simulink model "DeployableEMF"  (R2024a)
settings: Solver=FixedStepAuto  StartTime=0.0  StopTime=0  FixedStep=framePeriod_s  RelTol=1e-3
undefined symbols (not defined in the file): Aircraft, aircraftIC, AircraftModel, Avphi, DiscIntNeverNeededParam, EMF, EnableFF, EnableInputNoise, EnableRCHH, EnableSpeedHold, framePeriod_s, InitCond, Lv, Yv
libraries: simulink x14, simulink_extras x5
(part 1 of 2)
settings Model: Creator=zchen  LastModifiedBy=awalter
settings OptimizationCC: DefaultParameterBehavior=Inlined  GainParamInheritBuiltInType=on  UseFloatMulNetSlope=on  DefaultUnderspecifiedDataType=single  EnhancedBackFolding=on  PassReuseOutputArgsAs=Individual arguments  ZeroExternalMemoryAtStartup=off  ZeroInternalMemoryAtStartup=off  OptimizeBlockOrder=speed  DifferentSizesBufferReuse=on  OptimizationCustomize=off  EfficientTunableParamExpr=on
settings DebuggingCC: ParameterTunabilityLossMsg=error
settings HardwareCC: ProdLongLongMode=on
settings SFSimCC: MATLABDynamicMemAlloc=off
settings RTWCC: Description=Embedded Coder  SystemTargetFile=ert.tlc  GenCodeOnly=on  TemplateMakefile=ert_default_tmf  Toolchain=CMake  TargetLang=C++
settings CodeAppCC: ForceParamTrailComments=on  IgnoreCustomStorageClasses=off  OperatorAnnotations=on  SimulinkDataObjDesc=on  SFDataObjDesc=on  InsertBlockDesc=on
settings ERTTargetCC: TargetLangStandard=C++03 (ISO)  GenerateSampleERTMain=on  CodeInterfacePackaging=C++ class  InlinedParameterPlacement=NonHierarchical  RootIOFormat=Structure reference  ERTCustomFileTemplate=example_file_process.tlc

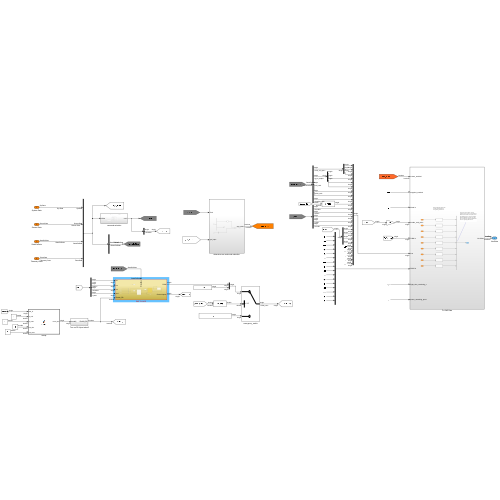
[thumbnail: Simulink's stored preview of the top-level diagram]
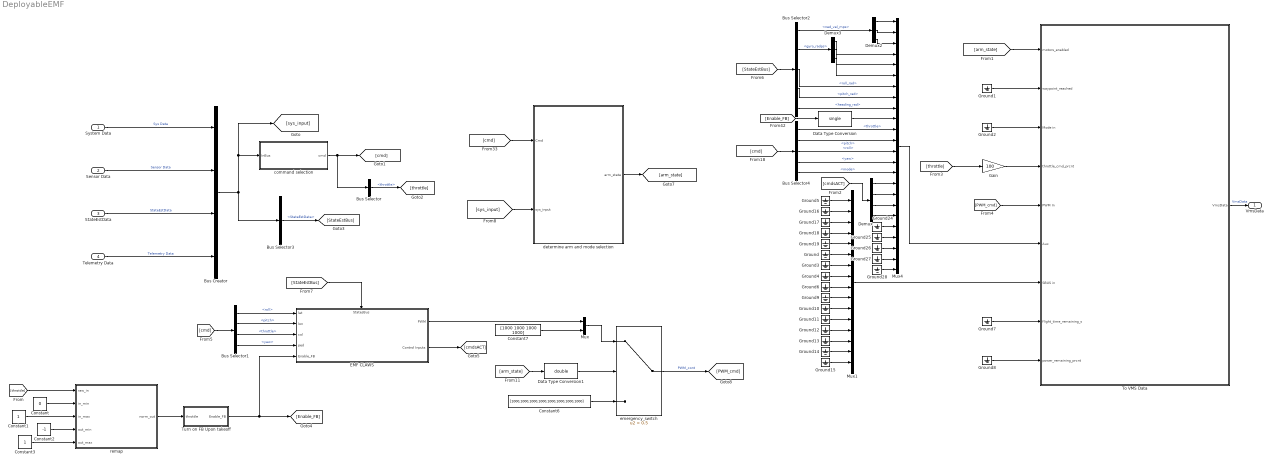
== system DeployableEMF ==
  System Data : Inport  OutDataTypeStr=Bus: SysData  SampleTime=framePeriod_s  BusOutputAsStruct=on
  Sensor Data : Inport  Port=2  OutDataTypeStr=Bus: SensorData  SampleTime=framePeriod_s  BusOutputAsStruct=on
  StateEstData : Inport  Port=3  OutDataTypeStr=Bus: StateEstData  SampleTime=framePeriod_s  BusOutputAsStruct=on
  Telemetry Data : Inport  Port=4  OutDataTypeStr=Bus: TelemData  SampleTime=framePeriod_s  BusOutputAsStruct=on
  Bus Creator : BusCreator  Inputs=4
  Bus Selector : BusSelector  OutputSignals=throttle
  Bus Selector1 : BusSelector  OutputSignals=roll,pitch,throttle,yaw
  Bus Selector2 : BusSelector  OutputSignals=bfs_ins.ned_vel_mps,bfs_ins.gyro_radps,bfs_ins.roll_rad,bfs_ins.pitch_rad,bfs_ins.heading_rad
  Bus Selector3 : BusSelector  OutputSignals=StateEstData
  Bus Selector4 : BusSelector  OutputSignals=throttle,pitch,roll,yaw,mode
  Constant : Constant  Value=0
  Constant1 : Constant
  Constant2 : Constant  Value=-1
  Constant3 : Constant
  Constant6 : Constant  Value=[1000,1000,1000,1000,1000,1000,1000,1000]  OutDataTypeStr=single
  Constant7 : Constant  Value=[1000 1000 1000 1000]  OutDataTypeStr=single
  Data Type Conversion : DataTypeConversion  OutDataTypeStr=single  SaturateOnIntegerOverflow=off  RndMeth=Floor
  Data Type Conversion1 : DataTypeConversion  OutDataTypeStr=double  SaturateOnIntegerOverflow=off  RndMeth=Floor
  Demux : Demux
  Demux2 : Demux  Outputs=3
  Demux3 : Demux  Outputs=3
  EMF CLAWS : Subsystem
      settings: PortSchema="{\"entries\":[{\"content\":{\"sides\":[{\"content\":{\"connectorIds\":[\"In1\",\"In2\",\"In3\",\"In4\",\"In5\"]},\"type\":\"ConnectorPlacement.EquallySpacedRectSide\",\"uuid\":\"fb2bd7fd-d988-4e33-8730-8c0f6eaa6827\"},{\"content\":{\"connectorIds\":[\"Out1\",\"Out2\"],\"side\":\"RIGHT\"},\"type\":\"ConnectorPlacement.EquallySpacedRectSide\",\"uuid\":\"7a7bb2dd-1c11-4f43-b871-d3aa786085a8\"},{\"content\":{\"connectorIds\":[\"In6\"],\"side\":\"TOP\"},\"type\":\"ConnectorPlacement.EquallySpacedRectSide\",\"uuid\":\"ea8fcfc4-ca21-4a8a-b475-95b355c5bc73\"},{\"content\":{\"side\":\"BOTTOM\"},\"type\":\"ConnectorPlacement.EquallySpacedRectSide\",\"uuid\":\"ba97ba4c-5167-4599-b94e-9748a5e0c732\"}]},\"type\":\"ConnectorPlacement.EquallySpacedConnector\",\"uuid\":\"d90d9832-6a61-4ee8-a098-cbdde4b4061b\"}],\"packageUris\":[\"http://schema.mathworks.com/mf0/Connector/R2020b\"],\"version\":\"1.0\"}"
  Gain : Gain  Gain=100
  Ground{,1..19,24..28} (25 alike) : Ground
  Mux : Mux  Inputs=2
  Mux1 : Mux  Inputs=16
  Mux4 : Mux  Inputs=24
  To VMS Data : Subsystem
  Turn on FB Upon takeoff : Subsystem
  command selection : Subsystem
  determine arm and mode selection : Subsystem
  emergency_switch : Switch  Criteria=u2 > Threshold  Threshold=0.5  SaturateOnIntegerOverflow=off  InputSameDT=off
  remap : MATLAB Function  TreatAsAtomicUnit=on
  VmsData : Outport  OutDataTypeStr=Bus: VmsData  SampleTime=framePeriod_s  BusOutputAsStruct=on
  wires:
  Turn on FB Upon takeoff/1(Enable_FB) -> [Enable_FB], EMF CLAWS/5(Enable_FB)
  Constant/1 -> remap/2(in_min)
  Ground7/1 -> To VMS Data/8(flight_time_remaining_s)
  [cmdsACT] -> Demux/1
  Ground/1 -> Mux1/6
  Bus Creator/1 -> Bus Selector3/1, [sys_input], command selection/1(InBus)
  Bus Selector1/3 -> EMF CLAWS/3(col)  "<throttle>"
  StateEstData/1 -> Bus Creator/3  "StateEstData"
  Mux4/1 -> To VMS Data/6(Aux)
  Bus Selector1/4 -> EMF CLAWS/4(ped)  "<yaw>"
  Ground14/1 -> Mux1/15
  Ground17/1 -> Mux1/3
  Bus Selector1/1 -> EMF CLAWS/1(lat)  "<roll>"
  Constant3/1 -> remap/5(out_max)
  Bus Selector1/2 -> EMF CLAWS/2(lon)  "<pitch>"
  [cmd] -> Bus Selector1/1
  determine arm and mode selection/1(arm_state) -> [arm_state]
  [arm_state] -> To VMS Data/1(motors_enabled)
  Ground1/1 -> To VMS Data/2(waypoint_reached)
  Bus Selector4/5 -> Mux4/15  "<mode>"
  [cmd] -> Bus Selector4/1
  Bus Selector4/4 -> Mux4/14  "<yaw>"
  [PWM_cmd] -> To VMS Data/5(PWM In)
  [Enable_FB] -> Data Type Conversion/1
  Ground9/1 -> Mux1/10
  Ground3/1 -> Mux1/7
  [throttle] -> Gain/1
  Ground16/1 -> Mux1/2
  Ground27/1 -> Mux4/23
  Ground28/1 -> Mux4/24
  Ground5/1 -> Mux1/1
  Demux/2 -> Mux4/17
  Ground4/1 -> Mux1/8
  command selection/1(cmd) -> Bus Selector/1, [cmd]
  Ground25/1 -> Mux4/21
  Constant1/1 -> remap/3(in_max)
  Data Type Conversion/1 -> Mux4/10
  Demux/4 -> Mux4/19
  Ground18/1 -> Mux1/4
  To VMS Data/1(VmsData) -> VmsData/1  "VmsData"
  EMF CLAWS/2(Control Inputs) -> [cmdsACT]
  Mux1/1 -> To VMS Data/7(SBUS in)
  Ground10/1 -> Mux1/11
  Ground19/1 -> Mux1/5
  Ground15/1 -> Mux1/16
  Demux/3 -> Mux4/18
  Bus Selector4/1 -> Mux4/11  "<throttle>"
  Ground2/1 -> To VMS Data/3(Mode in)
  Gain/1 -> To VMS Data/4(throttle_cmd_prcnt)
  Ground11/1 -> Mux1/12
  Bus Selector4/3 -> Mux4/13  "<roll>"
  System Data/1 -> Bus Creator/1  "Sys Data"
  [StateEstBus] -> EMF CLAWS/6(StatesBus)
  emergency_switch/1 -> [PWM_cmd]  "PWM_cont"
  Ground13/1 -> Mux1/14
  Telemetry Data/1 -> Bus Creator/4  "Telemetry Data"
  Constant2/1 -> remap/4(out_min)
  Data Type Conversion1/1 -> emergency_switch/2
  Constant7/1 -> Mux/2
  Demux/1 -> Mux4/16
  Ground8/1 -> To VMS Data/9(power_remaining_prcnt)
  Ground26/1 -> Mux4/22
  Bus Selector4/2 -> Mux4/12  "<pitch>"
  [cmd] -> determine arm and mode selection/1(Cmd)
  Ground6/1 -> Mux1/9
  [arm_state] -> Data Type Conversion1/1
  Sensor Data/1 -> Bus Creator/2  "Sensor Data"
  Ground24/1 -> Mux4/20
  Constant6/1 -> emergency_switch/3
  Bus Selector/1 -> [throttle]  "<throttle>"
  Mux/1 -> emergency_switch/1
  [throttle] -> remap/1(raw_in)
  Ground12/1 -> Mux1/13
  remap/1(norm_out) -> Turn on FB Upon takeoff/1(throttle)
  EMF CLAWS/1(PWM) -> Mux/1
  [sys_input] -> determine arm and mode selection/2(sys_input)
  Bus Selector3/1 -> [StateEstBus]  "<StateEstData>"
  Bus Selector2/5 -> Mux4/9  "<heading_rad>"
  Demux2/3 -> Mux4/3
  Bus Selector2/3 -> Mux4/7  "<roll_rad>"
  Demux2/2 -> Mux4/2
  Demux3/3 -> Mux4/6
  Demux2/1 -> Mux4/1
  Demux3/2 -> Mux4/5
  Demux3/1 -> Mux4/4
  Bus Selector2/1 -> Demux2/1  "<ned_vel_mps>"
  Bus Selector2/2 -> Demux3/1  "<gyro_radps>"
  [StateEstBus] -> Bus Selector2/1
  Bus Selector2/4 -> Mux4/8  "<pitch_rad>"

== system DeployableEMF/EMF CLAWS ==
  lat : Inport
  lon : Inport  Port=2
  col : Inport  Port=3
  ped : Inport  Port=4
  Enable_FB : Inport  Port=5
  StatesBus : Inport  Port=6
  ACAH Cmds & Spd Hold : Subsystem
      settings: PortSchema="{\"entries\":[{\"content\":{\"sides\":[{\"content\":{\"connectorIds\":[\"In1\",\"In2\"]},\"type\":\"ConnectorPlacement.EquallySpacedRectSide\",\"uuid\":\"c3aa03e9-ccb7-43c1-9798-8bf5432b2078\"},{\"content\":{\"connectorIds\":[\"Out1\",\"In3\"],\"side\":\"RIGHT\"},\"type\":\"ConnectorPlacement.EquallySpacedRectSide\",\"uuid\":\"89787a9d-9180-48b5-9998-cbe29e861495\"},{\"content\":{\"side\":\"TOP\"},\"type\":\"ConnectorPlacement.EquallySpacedRectSide\",\"uuid\":\"561bdc28-5c99-4c7e-b92e-eea3c95e9dce\"}]},\"type\":\"ConnectorPlacement.EquallySpacedConnector\",\"uuid\":\"f8321d21-0be0-47fc-a0ce-0477a72d6da9\"}],\"packageUris\":[\"http://schema.mathworks.com/mf0/Connector/R2020b\"],\"version\":\"1.0\"}"
  ACAH EMF1 : Subsystem
      settings: PortSchema="{\"entries\":[{\"content\":{\"sides\":[{\"content\":{\"connectorIds\":[\"In1\",\"In2\",\"In3\",\"In4\"]},\"type\":\"ConnectorPlacement.EquallySpacedRectSide\",\"uuid\":\"f0dc30a9-2643-4fce-a09e-da0b9dd6324b\"},{\"content\":{\"connectorIds\":[\"Out1\",\"Out2\",\"In5\"],\"side\":\"RIGHT\"},\"type\":\"ConnectorPlacement.EquallySpacedRectSide\",\"uuid\":\"f36ff2d8-c7c9-4ba3-92a3-b4ca37b19f9f\"},{\"content\":{\"side\":\"TOP\"},\"type\":\"ConnectorPlacement.EquallySpacedRectSide\",\"uuid\":\"7b352d47-5869-4cbf-a869-38e91cc0e44a\"},{\"content\":{\"side\":\"BOTTOM\"},\"type\":\"ConnectorPlacement.EquallySpacedRectSide\",\"uuid\":\"5fadfb50-1d15-4496-8b39-21c3867b197d\"}]},\"type\":\"ConnectorPlacement.EquallySpacedConnector\",\"uuid\":\"c5d3e032-086f-44da-ac5d-b4320e592dfa\"}],\"packageUris\":[\"http://schema.mathworks.com/mf0/Connector/R2020b\"],\"version\":\"1.0\"}"
  Mux : Mux
  PWM to Linear Model Inputs : Subsystem
  PWM : Outport
  Control Inputs : Outport  Port=2
  wires:
  StatesBus/1 -> ACAH Cmds & Spd Hold/3(StateEstBus), ACAH EMF1/4(StateEstBus)
  Mux/1 -> ACAH Cmds & Spd Hold/2(StickInputs), ACAH EMF1/1(cmdsStick)
  [Enable_FB] -> ACAH EMF1/2(Enable_FB)
  lat/1 -> Mux/1
  ACAH Cmds & Spd Hold/1(cmdsACAH) -> ACAH EMF1/3(cmdsACAH)
  [Enable_FB] -> ACAH Cmds & Spd Hold/1(Enable_FB)
  ped/1 -> Mux/4
  lon/1 -> Mux/2
  ACAH EMF1/1(PWM) -> PWM to Linear Model Inputs/1(PWM), PWM/1
  col/1 -> Mux/3
  Enable_FB/1 -> [Enable_FB]
  PWM to Linear Model Inputs/1(RotorSpeedsIn) -> ACAH EMF1/5(OmegasIn)
  ACAH EMF1/2(ControlInputs) -> Control Inputs/1

== system DeployableEMF/To VMS Data ==
  note: Cast to different data types to match with definition from global_definitions.h
  note: This is the bus creator. It acts similarly to the mux in Simulink but allows user match the inputs to the an arbitrary struct. This is useful to define interfaces. Check how this bus is matching with the VMS data struct in global_definitions.h
  motors_enabled : Inport
  waypoint_reached : Inport  Port=2
  Mode in : Inport  Port=3
  throttle_cmd_prcnt : Inport  Port=4
  PWM In : Inport  Port=5
  Aux : Inport  Port=6
  SBUS in : Inport  Port=7
  flight_time_remaining_s : Inport  Port=8
  power_remaining_prcnt : Inport  Port=9
  Bus Creator : BusCreator  Inputs=9  OutDataTypeStr=Bus: VmsData  NonVirtualBus=on
      settings: InheritFromInputs=off
  Cast : DataTypeConversion  OutDataTypeStr=int8  SaturateOnIntegerOverflow=off  RndMeth=Floor
  Cast To Boolean1 : DataTypeConversion  OutDataTypeStr=boolean  SaturateOnIntegerOverflow=off  RndMeth=Floor
  Cast To Boolean2 : DataTypeConversion  OutDataTypeStr=boolean  SaturateOnIntegerOverflow=off  RndMeth=Floor
  Cast To Single{,1..3} (4 alike) : DataTypeConversion  OutDataTypeStr=single  SaturateOnIntegerOverflow=off  RndMeth=Floor
  Cast1 : DataTypeConversion  OutDataTypeStr=int16  SaturateOnIntegerOverflow=off  RndMeth=Floor
  Cast2 : DataTypeConversion  OutDataTypeStr=int16  SaturateOnIntegerOverflow=off  RndMeth=Floor
  VmsData : Outport
  wires:
  Bus Creator/1 -> VmsData/1
  waypoint_reached/1 -> Cast To Boolean2/1  "advance_waypoint"
  motors_enabled/1 -> Cast To Boolean1/1  "motors_enabled"
  Mode in/1 -> Cast/1  "mode"
  SBUS in/1 -> Cast1/1  "sbus"
  PWM In/1 -> Cast2/1  "pwm"
  throttle_cmd_prcnt/1 -> Cast To Single1/1  "throttle_cmd_prcnt"
  Aux/1 -> Cast To Single3/1  "aux"
  Cast To Single2/1 -> Bus Creator/8  "power_remaining_prcnt"
  Cast To Single/1 -> Bus Creator/7  "flight_time_remaining_s"
  flight_time_remaining_s/1 -> Cast To Single/1  "flight_time_remaining_s"
  Cast To Boolean2/1 -> Bus Creator/1  "advance_waypoint"
  Cast To Boolean1/1 -> Bus Creator/2  "motors_enabled"
  Cast/1 -> Bus Creator/3  "mode"
  Cast1/1 -> Bus Creator/4  "sbus"
  Cast2/1 -> Bus Creator/5  "pwm"
  Cast To Single1/1 -> Bus Creator/6  "throttle_cmd_prcnt"
  power_remaining_prcnt/1 -> Cast To Single2/1  "power_remaining_prcnt"
  Cast To Single3/1 -> Bus Creator/9  "aux"

== system DeployableEMF/Turn on FB Upon takeoff ==
  throttle : Inport
  Constant3 : Constant
  Constant4 : Constant
  Constant5 : Constant  Value=0
  D Latch1 : simulink_extras/Flip Flops/D Latch
  Data Type Conversion2 : DataTypeConversion  SaturateOnIntegerOverflow=off  RndMeth=Floor
  Data Type Conversion3 : DataTypeConversion  SaturateOnIntegerOverflow=off  RndMeth=Floor
  Switch1 : Switch  Criteria=u2 > Threshold  Threshold=-0.2  SaturateOnIntegerOverflow=off  InputSameDT=off
  Terminator1 : Terminator
  Enable_FB : Outport
  wires:
  Constant4/1 -> Switch1/1
  Switch1/1 -> Data Type Conversion3/1
  D Latch1/1 -> Enable_FB/1
  throttle/1 -> Switch1/2
  Data Type Conversion3/1 -> D Latch1/2
  Constant3/1 -> Data Type Conversion2/1
  Data Type Conversion2/1 -> D Latch1/1
  D Latch1/2 -> Terminator1/1
  Constant5/1 -> Switch1/3

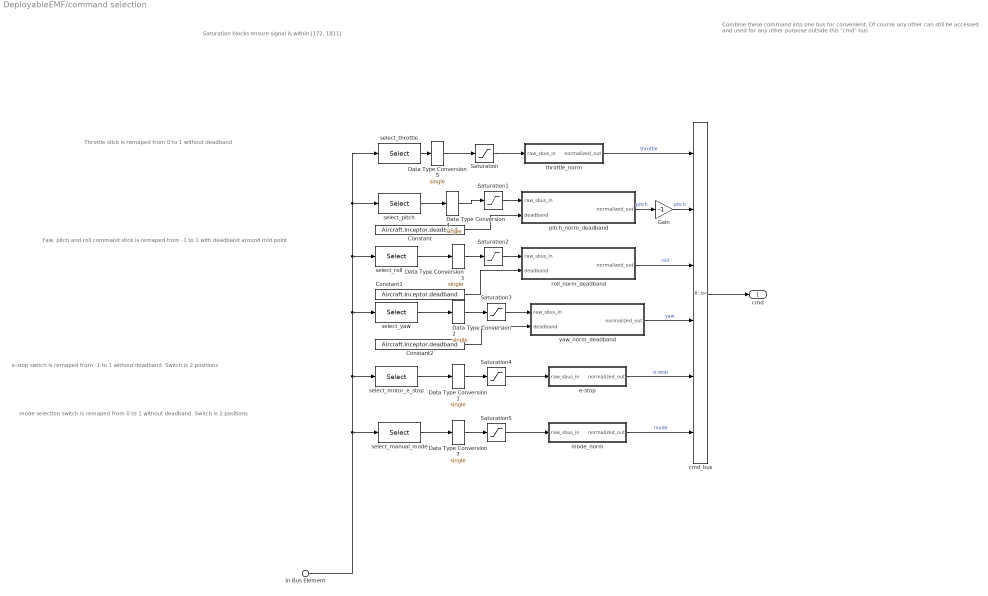
== system DeployableEMF/command selection ==
  note: Throttle stick is remaped from 0 to 1 without deadband
  note: Yaw, pitch and roll command stick is remaped from -1 to 1 with deadband around mid point
  note: e-stop switch is remaped from -1 to 1 without deadband. Switch is 2 positions
  note: mode selection switch is remaped from 0 to 1 without deadband. Switch is 2 positions
  note: Saturation blocks ensure signal is within [172, 1811]
  note: Combine these command into one bus for convenient. Of course any other can still be accessed and used for any other purpose outside this "cmd" bus
  In Bus Element : Inport  PortName=InBus  Element=Sensor Data.inceptor.ch
  Constant : Constant  Value=Aircraft.Inceptor.deadband  OutDataTypeStr=single
  Constant1 : Constant  Value=Aircraft.Inceptor.deadband  OutDataTypeStr=single
  Constant2 : Constant  Value=Aircraft.Inceptor.deadband  OutDataTypeStr=single
  Data Type Conversion{1..5,7} (6 alike) : DataTypeConversion  OutDataTypeStr=single  SaturateOnIntegerOverflow=off  RndMeth=Floor
  Gain : Gain  Gain=-1
  Saturation{,1..5} (6 alike) : Saturate  UpperLimit=1810  LowerLimit=174
  cmd_bus : BusCreator  Inputs=6
  e-stop : Subsystem
  mode_norm : Subsystem
  pitch_norm_deadband : Subsystem
  roll_norm_deadband : Subsystem
  select_manual_mode : Selector  IndexOptions=Index vector (dialog)  Indices=5  OutputSizes=1
  select_motor_e_stop : Selector  IndexOptions=Index vector (dialog)  Indices=8  OutputSizes=1
  select_pitch : Selector  IndexOptions=Index vector (dialog)  Indices=3  OutputSizes=1
  select_roll : Selector  IndexOptions=Index vector (dialog)  Indices=2  OutputSizes=1
  select_throttle : Selector  IndexOptions=Index vector (dialog)  Indices=1  OutputSizes=1
  select_yaw : Selector  IndexOptions=Index vector (dialog)  Indices=4  OutputSizes=1
  throttle_norm : Subsystem
  yaw_norm_deadband : Subsystem
  cmd : Outport
  wires:
  select_pitch/1 -> Data Type Conversion4/1
  select_yaw/1 -> Data Type Conversion2/1
  select_throttle/1 -> Data Type Conversion5/1
  cmd_bus/1 -> cmd/1
  Data Type Conversion5/1 -> Saturation/1
  select_roll/1 -> Data Type Conversion3/1
  Data Type Conversion1/1 -> Saturation4/1
  select_motor_e_stop/1 -> Data Type Conversion1/1
  Data Type Conversion7/1 -> Saturation5/1
  select_manual_mode/1 -> Data Type Conversion7/1
  Data Type Conversion2/1 -> Saturation3/1
  Constant2/1 -> yaw_norm_deadband/2(deadband)
  throttle_norm/1(normalized_out) -> cmd_bus/1  "throttle"
  roll_norm_deadband/1(normalized_out) -> cmd_bus/3  "roll"
  pitch_norm_deadband/1(normalized_out) -> Gain/1  "pitch"
  Data Type Conversion4/1 -> Saturation1/1
  Constant/1 -> pitch_norm_deadband/2(deadband)
  Constant1/1 -> roll_norm_deadband/2(deadband)
  Data Type Conversion3/1 -> Saturation2/1
  yaw_norm_deadband/1(normalized_out) -> cmd_bus/4  "yaw"
  e-stop/1(normalized_out) -> cmd_bus/5  "e-stop"
  mode_norm/1(normalized_out) -> cmd_bus/6  "mode"
  In Bus Element/1 -> select_roll/1, select_throttle/1, select_pitch/1, select_yaw/1, select_motor_e_stop/1, select_manual_mode/1
  Saturation/1 -> throttle_norm/1(raw_sbus_in)
  Saturation2/1 -> roll_norm_deadband/1(raw_sbus_in)
  Saturation3/1 -> yaw_norm_deadband/1(raw_sbus_in)
  Saturation4/1 -> e-stop/1(raw_sbus_in)
  Saturation5/1 -> mode_norm/1(raw_sbus_in)
  Saturation1/1 -> pitch_norm_deadband/1(raw_sbus_in)
  Gain/1 -> cmd_bus/2  "pitch"

== system DeployableEMF/determine arm and mode selection ==
  Cmd : Inport
  sys_input : Inport  Port=2
  AND : Logic  IconShape=distinctive  AllPortsSameDT=off  OutDataTypeStr=boolean
  Bus Selector : BusSelector  OutputSignals=StateEstData.bfs_ins.initialized
  Bus Selector1 : BusSelector  OutputSignals=mode,throttle
  Compare To Constant1 : simulink/Logic and Bit Operations/Compare To Constant  relop=>  const=0.5  OutDataTypeStr=boolean
  Terminator : Terminator
  arm_state : Outport
  wires:
  Cmd/1 -> Bus Selector1/1
  Bus Selector1/2 -> Terminator/1  "<throttle>"
  sys_input/1 -> Bus Selector/1
  Compare To Constant1/1 -> AND/1
  AND/1 -> arm_state/1
  Bus Selector1/1 -> Compare To Constant1/1  "<mode>"
  Bus Selector/1 -> AND/2  "<initialized>"

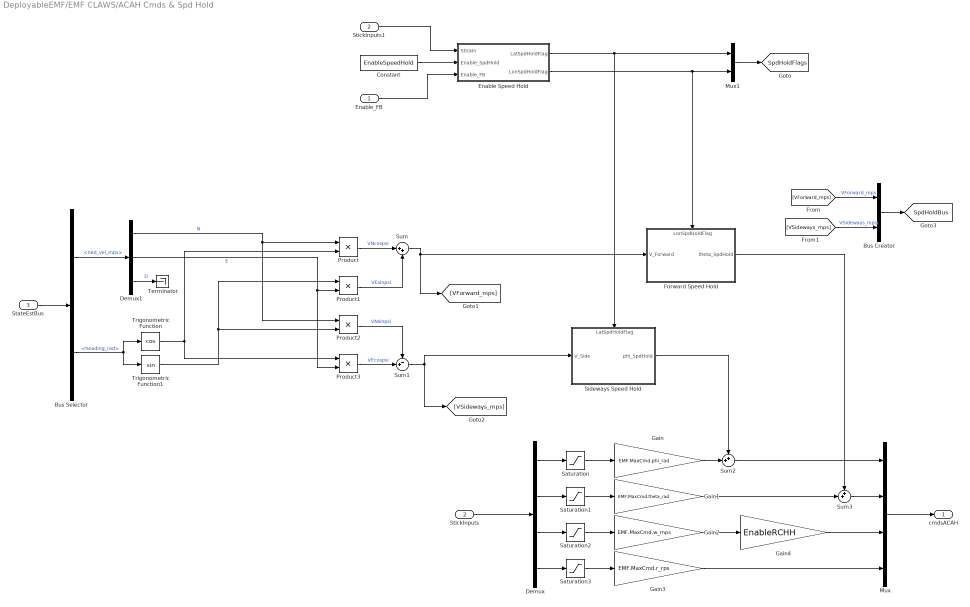
== system DeployableEMF/EMF CLAWS/ACAH Cmds & Spd Hold ==
  Enable_FB : Inport
  StickInputs : Inport  Port=2
  StateEstBus : Inport  Port=3
  Bus Creator : BusCreator  Inputs=2
  Bus Selector : BusSelector  OutputSignals=bfs_ins.ned_vel_mps,bfs_ins.heading_rad
  Constant : Constant  Value=EnableSpeedHold
  Demux : Demux
  Demux1 : Demux  Outputs=3
  Enable Speed Hold : Subsystem
  Forward Speed Hold : Subsystem
      settings: PortSchema="{\"entries\":[{\"content\":{\"sides\":[{\"content\":{\"connectorIds\":[\"In1\"]},\"type\":\"ConnectorPlacement.EquallySpacedRectSide\",\"uuid\":\"787a0d40-d54a-40fd-80f9-efd334690e34\"},{\"content\":{\"connectorIds\":[\"Out1\"],\"side\":\"RIGHT\"},\"type\":\"ConnectorPlacement.EquallySpacedRectSide\",\"uuid\":\"f6a8c8e2-752b-42ff-b4f2-32f20fdea40d\"},{\"content\":{\"connectorIds\":[\"In2\"],\"side\":\"TOP\"},\"type\":\"ConnectorPlacement.EquallySpacedRectSide\",\"uuid\":\"415bab51-e904-4948-b139-fad0363c569f\"},{\"content\":{\"side\":\"BOTTOM\"},\"type\":\"ConnectorPlacement.EquallySpacedRectSide\",\"uuid\":\"fe1710f6-98f7-4914-bba4-54f9a2ec34d8\"}]},\"type\":\"ConnectorPlacement.EquallySpacedConnector\",\"uuid\":\"a4ae154f-8926-4c51-a0ea-11671019ffb8\"}],\"packageUris\":[\"http://schema.mathworks.com/mf0/Connector/R2020b\"],\"version\":\"1.0\"}"
  Gain : Gain  Gain=EMF.MaxCmd.phi_rad
  Gain1 : Gain  Gain=EMF.MaxCmd.theta_rad
  Gain2 : Gain  Gain=EMF.MaxCmd.w_mps
  Gain3 : Gain  Gain=EMF.MaxCmd.r_rps
  Gain4 : Gain  Gain=EnableRCHH
  Mux : Mux
  Mux1 : Mux  Inputs=2
  Product{,1..3} (4 alike) : Product
  Saturation{,1..3} (4 alike) : Saturate  UpperLimit=1  LowerLimit=-1
  Sideways Speed Hold : Subsystem
      settings: PortSchema="{\"entries\":[{\"content\":{\"sides\":[{\"content\":{\"connectorIds\":[\"In1\"]},\"type\":\"ConnectorPlacement.EquallySpacedRectSide\",\"uuid\":\"787a0d40-d54a-40fd-80f9-efd334690e34\"},{\"content\":{\"connectorIds\":[\"Out1\"],\"side\":\"RIGHT\"},\"type\":\"ConnectorPlacement.EquallySpacedRectSide\",\"uuid\":\"f6a8c8e2-752b-42ff-b4f2-32f20fdea40d\"},{\"content\":{\"connectorIds\":[\"In2\"],\"side\":\"TOP\"},\"type\":\"ConnectorPlacement.EquallySpacedRectSide\",\"uuid\":\"415bab51-e904-4948-b139-fad0363c569f\"}]},\"type\":\"ConnectorPlacement.EquallySpacedConnector\",\"uuid\":\"a4ae154f-8926-4c51-a0ea-11671019ffb8\"}],\"packageUris\":[\"http://schema.mathworks.com/mf0/Connector/R2020b\"],\"version\":\"1.0\"}"
  StickInputs1 : InportShadow  Port=2
  Sum : Sum  Inputs=|++
  Sum1 : Sum  Inputs=-+|
  Sum2 : Sum  Inputs=++|
  Sum3 : Sum  Inputs=++|
  Terminator : Terminator
  Trigonometric Function : Trigonometry  Operator=cos
  Trigonometric Function1 : Trigonometry
  cmdsACAH : Outport
  tag scope: SpdHoldBus=global, SpdHoldFlags=global
  wires:
  Demux/1 -> Saturation/1
  Demux/2 -> Saturation1/1
  Demux/3 -> Saturation2/1
  Demux/4 -> Saturation3/1
  Saturation/1 -> Gain/1
  Saturation1/1 -> Gain1/1
  Saturation2/1 -> Gain2/1
  Saturation3/1 -> Gain3/1
  Gain2/1 -> Gain4/1
  Gain3/1 -> Mux/4
  Sum3/1 -> Mux/2
  Gain/1 -> Sum2/2
  StateEstBus/1 -> Bus Selector/1
  Mux/1 -> cmdsACAH/1
  StickInputs/1 -> Demux/1
  Demux1/1 -> Product/1, Product2/1  "N"
  Demux1/2 -> Product3/2, Product1/2  "E"
  Bus Selector/2 -> Trigonometric Function1/1, Trigonometric Function/1  "<heading_rad>"
  Trigonometric Function/1 -> Product/2, Product3/1
  Trigonometric Function1/1 -> Product2/2, Product1/1
  Product/1 -> Sum/1  "VNcospsi"
  Product2/1 -> Sum1/1  "VNsinpsi"
  Product3/1 -> Sum1/2  "VEcospsi"
  Product1/1 -> Sum/2  "VEsinpsi"
  Sum1/1 -> [VSideways_mps], Sideways Speed Hold/1(V_Side)
  Enable Speed Hold/2(LonSpdHoldFlag) -> Forward Speed Hold/2(LonSpdHoldFlag), Mux1/2
  Sum2/1 -> Mux/1
  Sideways Speed Hold/1(phi_SpdHold) -> Sum2/1
  Gain1/1 -> Sum3/2
  Forward Speed Hold/1(theta_SpdHold) -> Sum3/1
  Sum/1 -> [VForward_mps], Forward Speed Hold/1(V_Forward)
  StickInputs1/1 -> Enable Speed Hold/1(StickIn)
  Enable_FB/1 -> Enable Speed Hold/3(Enable_FB)
  Constant/1 -> Enable Speed Hold/2(Enable_SpdHold)
  Mux1/1 -> [SpdHoldFlags]
  Enable Speed Hold/1(LatSpdHoldFlag) -> Mux1/1, Sideways Speed Hold/2(LatSpdHoldFlag)
  Gain4/1 -> Mux/3
  [VForward_mps] -> Bus Creator/1  "VForward_mps"
  [VSideways_mps] -> Bus Creator/2  "VSideways_mps"
  Bus Creator/1 -> [SpdHoldBus]
  Bus Selector/1 -> Demux1/1  "<ned_vel_mps>"
  Demux1/3 -> Terminator/1  "D"

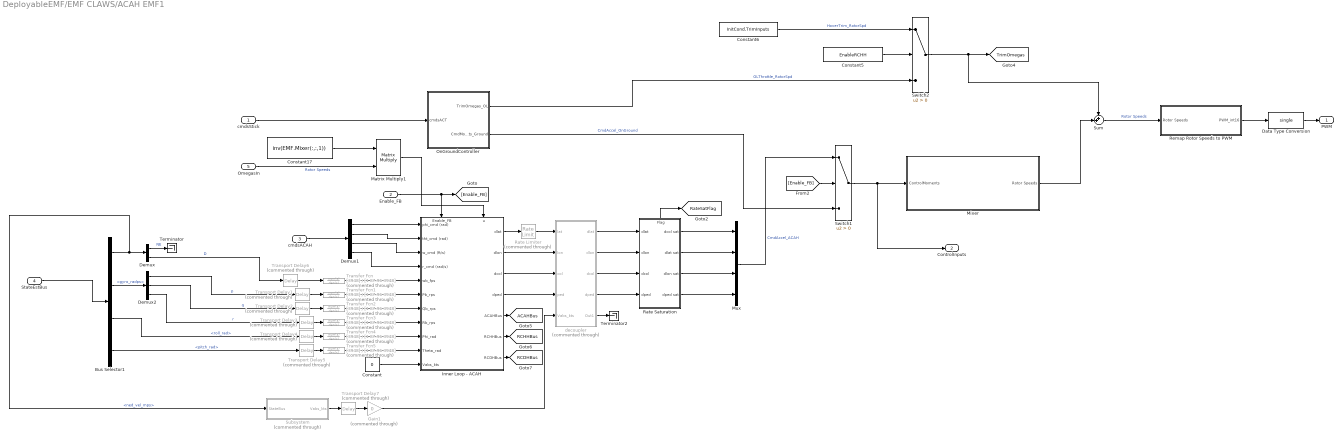
== system DeployableEMF/EMF CLAWS/ACAH EMF1 ==
  cmdsStick : Inport
  Enable_FB : Inport  Port=2
  cmdsACAH : Inport  Port=3
  StateEstBus : Inport  Port=4
  OmegasIn : Inport  Port=5
  Bus Selector1 : BusSelector  OutputSignals=bfs_ins.ned_vel_mps,bfs_ins.gyro_radps,bfs_ins.roll_rad,bfs_ins.pitch_rad
  Constant : Constant  Value=0
  Constant17 : Constant  Value=inv(EMF.Mixer(:,:,1))
  Constant5 : Constant  Value=EnableRCHH
  Constant6 : Constant  Value=InitCond.TrimInputs
  Data Type Conversion : DataTypeConversion  OutDataTypeStr=single  SaturateOnIntegerOverflow=off  RndMeth=Floor
  Demux : Demux  Outputs=[2 1]
  Demux1 : Demux
  Demux2 : Demux  Outputs=3
  Gain1 : Gain  Commented=through  Gain=0
  Inner Loop - ACAH : Subsystem
      settings: PortSchema="{\"entries\":[{\"content\":{\"sides\":[{\"content\":{\"connectorIds\":[\"In1\",\"In2\",\"In3\",\"In4\",\"In5\",\"In6\",\"In7\",\"In8\",\"In9\",\"In10\",\"In11\"]},\"type\":\"ConnectorPlacement.EquallySpacedRectSide\",\"uuid\":\"367df013-e636-4493-878e-e6ce959f1a3d\"},{\"content\":{\"connectorIds\":[\"Out1\",\"Out2\",\"Out3\",\"Out4\",\"Out5\",\"Out6\",\"Out7\"],\"side\":\"RIGHT\"},\"type\":\"ConnectorPlacement.EquallySpacedRectSide\",\"uuid\":\"2f0f56b3-a260-4d27-a040-b71c87136d50\"},{\"content\":{\"connectorIds\":[\"In12\",\"In13\"],\"side\":\"TOP\"},\"type\":\"ConnectorPlacement.EquallySpacedRectSide\",\"uuid\":\"e1b8f7b8-0af1-4704-8561-c2315c417309\"}]},\"type\":\"ConnectorPlacement.EquallySpacedConnector\",\"uuid\":\"a38a38a3-a4a0-48d0-95d7-3f832c6f2a49\"}],\"packageUris\":[\"http://schema.mathworks.com/mf0/Connector/R2020b\"],\"version\":\"1.0\"}"
  Matrix Multiply1 : Product  Multiplication=Matrix(*)
  Mixer : Subsystem
  Mux : Mux
  OnGroundController : Subsystem
  Rate Limiter : RateLimiter  Commented=through  RisingSlewLimit=20  FallingSlewLimit=-20  SampleTimeMode=inherited
  Rate Saturation : Subsystem
      settings: PortSchema="{\"entries\":[{\"content\":{\"sides\":[{\"content\":{\"connectorIds\":[\"In1\",\"In2\",\"In3\",\"In4\"]},\"type\":\"ConnectorPlacement.EquallySpacedRectSide\",\"uuid\":\"375e93bc-5dae-470f-aab8-5ad70d1e1811\"},{\"content\":{\"connectorIds\":[\"Out1\",\"Out2\",\"Out3\",\"Out4\"],\"side\":\"RIGHT\"},\"type\":\"ConnectorPlacement.EquallySpacedRectSide\",\"uuid\":\"dbec4a51-e0b1-4904-ace9-4cee9241c20c\"},{\"content\":{\"connectorIds\":[\"Out5\"],\"side\":\"TOP\"},\"type\":\"ConnectorPlacement.EquallySpacedRectSide\",\"uuid\":\"b9bfaa38-a6cc-462a-b2b2-3910847dbe04\"}]},\"type\":\"ConnectorPlacement.EquallySpacedConnector\",\"uuid\":\"703f1ade-6510-4079-b70f-cf26949c7e50\"}],\"packageUris\":[\"http://schema.mathworks.com/mf0/Connector/R2020b\"],\"version\":\"1.0\"}"
  Remap Rotor Speeds to PWM : Subsystem
  Subsystem : Subsystem  Commented=through
  Sum : Sum  Inputs=++|
  Switch1 : Switch  Criteria=u2 > Threshold  SaturateOnIntegerOverflow=off  InputSameDT=off
  Switch2 : Switch  Criteria=u2 > Threshold  SaturateOnIntegerOverflow=off  InputSameDT=off
  Terminator : Terminator
  Terminator2 : Terminator
  Transfer Fcn{,1..5} (6 alike) : TransferFcn  Commented=through  Numerator=[3948]  Denominator=[1 87.96 3948]
  Transport Delay{1..7} (7 alike) : TransportDelay  Commented=through  DelayTime=.02
  decoupler : Subsystem  Commented=through
  PWM : Outport
  ControlInputs : Outport  Port=2
  tag scope: ACAHBus=global, RCDHBus=global, RCHHBus=global, RateSatFlag=global, TrimOmegas=global
  wires:
  Rate Limiter/1 -> decoupler/1(lat)
  Inner Loop - ACAH/3(dcol) -> decoupler/3(col)
  Demux1/3 -> Inner Loop - ACAH/3(w_cmd (ft/s))
  Demux1/2 -> Inner Loop - ACAH/2(tht_cmd (rad))
  decoupler/5(Out1) -> Terminator2/1
  Transport Delay1/1 -> Transfer Fcn1/1
  Transport Delay3/1 -> Transfer Fcn3/1
  Transfer Fcn4/1 -> Inner Loop - ACAH/9(Phi_rad)
  Demux1/4 -> Inner Loop - ACAH/4(r_cmd (rad/s))
  Enable_FB/1 -> [Enable_FB], Inner Loop - ACAH/12(Enable_FB)
  Transfer Fcn/1 -> Inner Loop - ACAH/5(wb_fps)
  Inner Loop - ACAH/1(dlat) -> Rate Limiter/1
  Transfer Fcn5/1 -> Inner Loop - ACAH/10(Theta_rad)
  Transfer Fcn3/1 -> Inner Loop - ACAH/8(Rb_rps)
  Demux/2 -> Transport Delay6/1  "D"
  Demux2/1 -> Transport Delay1/1  "p"
  Subsystem/1(Vabs_kts) -> Transport Delay7/1
  Transport Delay6/1 -> Transfer Fcn/1
  Transport Delay5/1 -> Transfer Fcn5/1
  Demux2/3 -> Transport Delay3/1  "r"
  cmdsACAH/1 -> Demux1/1
  Transport Delay2/1 -> Transfer Fcn2/1
  Inner Loop - ACAH/4(dped) -> decoupler/4(ped)
  Transfer Fcn1/1 -> Inner Loop - ACAH/6(Pb_rps)
  Inner Loop - ACAH/2(dlon) -> decoupler/2(lon)
  StateEstBus/1 -> Bus Selector1/1
  Transport Delay4/1 -> Transfer Fcn4/1
  Transport Delay7/1 -> Gain1/1
  Demux1/1 -> Inner Loop - ACAH/1(phi_cmd (rad))
  Transfer Fcn2/1 -> Inner Loop - ACAH/7(Qb_rps)
  Demux2/2 -> Transport Delay2/1  "q"
  Switch2/1 -> [TrimOmegas], Sum/1
  cmdsStick/1 -> OnGroundController/1(cmdsACT)
  Mux/1 -> Switch1/1  "CmdAccel_ACAH"
  [Enable_FB] -> Switch1/2
  OnGroundController/2(CmdMoments_Ground) -> Switch1/3  "CmdAccel_OnGround"
  Constant5/1 -> Switch2/2
  OnGroundController/1(TrimOmegas_OL) -> Switch2/3  "OLThrottle_RotorSpd"
  Constant6/1 -> Switch2/1  "HoverTrim_RotorSpd"
  Gain1/1 -> decoupler/5(Vabs_kts)
  decoupler/1(dlat) -> Rate Saturation/1(dlat)
  decoupler/2(dlon) -> Rate Saturation/2(dlon)
  decoupler/3(dcol) -> Rate Saturation/3(dcol)
  decoupler/4(dped) -> Rate Saturation/4(dped)
  Rate Saturation/1(dcol sat) -> Mux/1
  Rate Saturation/2(dlat sat) -> Mux/2
  Rate Saturation/3(dlon sat) -> Mux/3
  Rate Saturation/4(dped sat) -> Mux/4
  Rate Saturation/5(Flag) -> [RateSatFlag]
  OmegasIn/1 -> Matrix Multiply1/2  "Rotor Speeds"
  Constant17/1 -> Matrix Multiply1/1
  Matrix Multiply1/1 -> Inner Loop - ACAH/13(u)
  Mixer/1(Rotor Speeds) -> Sum/2
  Switch1/1 -> ControlInputs/1, Mixer/1(ControlMoments)
  Inner Loop - ACAH/5(ACAHBus) -> [ACAHBus]
  Inner Loop - ACAH/6(RCHHBus) -> [RCHHBus]
  Inner Loop - ACAH/7(RCDHBus) -> [RCDHBus]
  Constant/1 -> Inner Loop - ACAH/11(Vabs_kts)
  Bus Selector1/1 -> Demux/1, Subsystem/1(StateBus)  "<ned_vel_mps>"
  Demux/1 -> Terminator/1  "NE"
  Bus Selector1/2 -> Demux2/1  "<gyro_radps>"
  Bus Selector1/3 -> Transport Delay4/1  "<roll_rad>"
  Bus Selector1/4 -> Transport Delay5/1  "<pitch_rad>"
  Sum/1 -> Remap Rotor Speeds to PWM/1(Rotor Speeds)  "Rotor Speeds"
  Remap Rotor Speeds to PWM/1(PWM_int16) -> Data Type Conversion/1
  Data Type Conversion/1 -> PWM/1

== system DeployableEMF/EMF CLAWS/PWM to Linear Model Inputs ==
  PWM : Inport
  Constant1 : Constant  Value=AircraftModel.MaxPWMLimit*ones(1,4)
  Constant11 : Constant  Value=AircraftModel.MinOmegaLimit
  Constant13 : Constant  Value=InitCond.TrimInputs
  Constant2 : Constant  Value=AircraftModel.MaxOmegaLimit
  Constant9 : Constant  Value=AircraftModel.MinPWMLimit*ones(1,4)
  Data Type Conversion1 : DataTypeConversion  OutDataTypeStr=double  SaturateOnIntegerOverflow=off  RndMeth=Floor
  Sum2 : Sum  Inputs=-+|
  remap : MATLAB Function  TreatAsAtomicUnit=on
  RotorSpeedsIn : Outport
  wires:
  Data Type Conversion1/1 -> remap/1(norm_in)
  Constant9/1 -> remap/2(in_min)
  Constant1/1 -> remap/3(in_max)
  Constant11/1 -> remap/4(out_min)
  Constant2/1 -> remap/5(out_max)
  remap/1(raw_out) -> Sum2/2
  Sum2/1 -> RotorSpeedsIn/1
  Constant13/1 -> Sum2/1
  PWM/1 -> Data Type Conversion1/1

== system DeployableEMF/command selection/e-stop ==
  raw_sbus_in : Inport
  Constant : Constant  Value=174  OutDataTypeStr=single
  Constant1 : Constant  Value=0  OutDataTypeStr=single
  Constant2 : Constant  OutDataTypeStr=single
  Constant3 : Constant  Value=1811  OutDataTypeStr=single
  remap : MATLAB Function  TreatAsAtomicUnit=on
  normalized_out : Outport
  wires:
  Constant2/1 -> remap/5(out_max)
  Constant1/1 -> remap/4(out_min)
  Constant3/1 -> remap/3(in_max)
  Constant/1 -> remap/2(in_min)
  remap/1(norm_out) -> normalized_out/1
  raw_sbus_in/1 -> remap/1(raw_in)

== system DeployableEMF/command selection/mode_norm ==
  raw_sbus_in : Inport
  Constant : Constant  Value=174  OutDataTypeStr=single
  Constant1 : Constant  Value=0  OutDataTypeStr=single
  Constant2 : Constant  OutDataTypeStr=single
  Constant3 : Constant  Value=1810  OutDataTypeStr=single
  remap : MATLAB Function  TreatAsAtomicUnit=on
  normalized_out : Outport
  wires:
  raw_sbus_in/1 -> remap/1(raw_in)
  remap/1(norm_out) -> normalized_out/1
  Constant/1 -> remap/2(in_min)
  Constant3/1 -> remap/3(in_max)
  Constant1/1 -> remap/4(out_min)
  Constant2/1 -> remap/5(out_max)

== system DeployableEMF/command selection/pitch_norm_deadband ==
  raw_sbus_in : Inport
  deadband : Inport  Port=2
  Constant : Constant  Value=174  OutDataTypeStr=single
  Constant1 : Constant  Value=-1  OutDataTypeStr=single
  Constant2 : Constant  OutDataTypeStr=single
  Constant3 : Constant  Value=1810  OutDataTypeStr=single
  remap_with_deadband : MATLAB Function  TreatAsAtomicUnit=on
  normalized_out : Outport
  wires:
  deadband/1 -> remap_with_deadband/6(deadband)
  Constant2/1 -> remap_with_deadband/5(out_max)
  Constant1/1 -> remap_with_deadband/4(out_min)
  Constant3/1 -> remap_with_deadband/3(in_max)
  Constant/1 -> remap_with_deadband/2(in_min)
  remap_with_deadband/1(norm_out) -> normalized_out/1
  raw_sbus_in/1 -> remap_with_deadband/1(raw_in)

== system DeployableEMF/command selection/roll_norm_deadband ==
  raw_sbus_in : Inport
  deadband : Inport  Port=2
  Constant : Constant  Value=174  OutDataTypeStr=single
  Constant1 : Constant  Value=-1  OutDataTypeStr=single
  Constant2 : Constant  OutDataTypeStr=single
  Constant3 : Constant  Value=1810  OutDataTypeStr=single
  remap_with_deadband : MATLAB Function  TreatAsAtomicUnit=on
  normalized_out : Outport
  wires:
  deadband/1 -> remap_with_deadband/6(deadband)
  Constant2/1 -> remap_with_deadband/5(out_max)
  Constant1/1 -> remap_with_deadband/4(out_min)
  Constant3/1 -> remap_with_deadband/3(in_max)
  Constant/1 -> remap_with_deadband/2(in_min)
  remap_with_deadband/1(norm_out) -> normalized_out/1
  raw_sbus_in/1 -> remap_with_deadband/1(raw_in)

== system DeployableEMF/command selection/throttle_norm ==
  raw_sbus_in : Inport
  Constant : Constant  Value=174  OutDataTypeStr=single
  Constant1 : Constant  Value=0  OutDataTypeStr=single
  Constant2 : Constant  OutDataTypeStr=single
  Constant3 : Constant  Value=1810  OutDataTypeStr=single
  remap : MATLAB Function  TreatAsAtomicUnit=on
  normalized_out : Outport
  wires:
  raw_sbus_in/1 -> remap/1(raw_in)
  remap/1(norm_out) -> normalized_out/1
  Constant/1 -> remap/2(in_min)
  Constant3/1 -> remap/3(in_max)
  Constant1/1 -> remap/4(out_min)
  Constant2/1 -> remap/5(out_max)

== system DeployableEMF/command selection/yaw_norm_deadband ==
  raw_sbus_in : Inport
  deadband : Inport  Port=2
  Constant : Constant  Value=174  OutDataTypeStr=single
  Constant1 : Constant  Value=-1  OutDataTypeStr=single
  Constant2 : Constant  OutDataTypeStr=single
  Constant3 : Constant  Value=1810  OutDataTypeStr=single
  remap_with_deadband : MATLAB Function  TreatAsAtomicUnit=on
  normalized_out : Outport
  wires:
  raw_sbus_in/1 -> remap_with_deadband/1(raw_in)
  remap_with_deadband/1(norm_out) -> normalized_out/1
  Constant/1 -> remap_with_deadband/2(in_min)
  Constant3/1 -> remap_with_deadband/3(in_max)
  Constant1/1 -> remap_with_deadband/4(out_min)
  Constant2/1 -> remap_with_deadband/5(out_max)
  deadband/1 -> remap_with_deadband/6(deadband)

== system DeployableEMF/EMF CLAWS/ACAH Cmds & Spd Hold/Enable Speed Hold ==
  StickIn : Inport
  Enable_SpdHold : Inport  Port=2
  Enable_FB : Inport  Port=3
  Abs : Abs  SaturateOnIntegerOverflow=off
  Abs1 : Abs  SaturateOnIntegerOverflow=off
  Constant : Constant  Value=0
  Constant1 : Constant
  Constant2 : Constant  Value=0
  Constant3 : Constant
  Deadzone : Switch  Criteria=u2 > Threshold  Threshold=0.1  SaturateOnIntegerOverflow=off  InputSameDT=off
  Deadzone1 : Switch  Criteria=u2 > Threshold  Threshold=0.1  SaturateOnIntegerOverflow=off  InputSameDT=off
  Demux : Demux
  Logical Operator : Logic  Inputs=3  AllPortsSameDT=off  OutDataTypeStr=boolean
  Logical Operator1 : Logic  Inputs=3  AllPortsSameDT=off  OutDataTypeStr=boolean
  Terminator : Terminator
  Terminator1 : Terminator
  LatSpdHoldFlag : Outport
  LonSpdHoldFlag : Outport  Port=2
  wires:
  Demux/4 -> Terminator1/1
  Demux/1 -> Abs/1
  Demux/3 -> Terminator/1
  Demux/2 -> Abs1/1
  StickIn/1 -> Demux/1
  Abs/1 -> Deadzone/2
  Abs1/1 -> Deadzone1/2
  Constant/1 -> Deadzone1/1
  Constant1/1 -> Deadzone1/3
  Constant2/1 -> Deadzone/1
  Constant3/1 -> Deadzone/3
  Deadzone/1 -> Logical Operator/1
  Deadzone1/1 -> Logical Operator1/1
  Enable_SpdHold/1 -> Logical Operator/2, Logical Operator1/2
  Logical Operator/1 -> LatSpdHoldFlag/1
  Logical Operator1/1 -> LonSpdHoldFlag/1
  Enable_FB/1 -> Logical Operator/3, Logical Operator1/3

== system DeployableEMF/EMF CLAWS/ACAH Cmds & Spd Hold/Forward Speed Hold ==
  note: Reset Integrator when speed hold turns on
  V_Forward : Inport
  LonSpdHoldFlag : Inport  Port=2
  Constant : Constant  Value=0.5
  Discrete-Time Integrator : DiscreteIntegrator  ExternalReset=rising  SampleTime=-1  ICPrevOutput=DiscIntNeverNeededParam  ICPrevScaledInput=DiscIntNeverNeededParam
  Gain : Gain  Gain=-1
  Gain1 : Gain  Gain=-1
  IntRat_V_F : Gain  Gain=0.08
  LonSpdHoldFlag1 : InportShadow  Port=2
  P_V_F : Gain  Gain=5*pi/180
  Product : Product
  Sum : Sum  Inputs=|+-
  Sum2 : Sum  Inputs=|++
  theta_SpdHold : Outport
  wires:
  Sum2/1 -> Gain1/1
  P_V_F/1 -> IntRat_V_F/1, Sum2/1
  IntRat_V_F/1 -> Discrete-Time Integrator/1
  Discrete-Time Integrator/1 -> Sum2/2
  V_Forward/1 -> Gain/1
  Gain/1 -> P_V_F/1  "V_Forward_Error"
  Product/1 -> theta_SpdHold/1
  Sum/1 -> Discrete-Time Integrator/2
  LonSpdHoldFlag/1 -> Sum/1
  Constant/1 -> Sum/2
  Gain1/1 -> Product/2
  LonSpdHoldFlag1/1 -> Product/1

== system DeployableEMF/EMF CLAWS/ACAH Cmds & Spd Hold/Sideways Speed Hold ==
  note: Reset Integrator when speed hold turns on
  V_Side : Inport
  LatSpdHoldFlag : Inport  Port=2
  Constant : Constant  Value=0.5
  Discrete-Time Integrator : DiscreteIntegrator  ExternalReset=rising  SampleTime=-1  ICPrevOutput=DiscIntNeverNeededParam  ICPrevScaledInput=DiscIntNeverNeededParam
  Gain : Gain  Gain=-1
  IntRat_V_S : Gain  Gain=0.08
  LatSpdHoldFlag1 : InportShadow  Port=2
  P_V_S : Gain  Gain=10*pi/180
  Product : Product
  Sum : Sum  Inputs=|+-
  Sum2 : Sum  Inputs=|++
  phi_SpdHold : Outport
  wires:
  Gain/1 -> P_V_S/1  "V_Side_Error"
  V_Side/1 -> Gain/1
  Discrete-Time Integrator/1 -> Sum2/2
  IntRat_V_S/1 -> Discrete-Time Integrator/1
  P_V_S/1 -> Sum2/1, IntRat_V_S/1
  Product/1 -> phi_SpdHold/1
  Sum/1 -> Discrete-Time Integrator/2
  Constant/1 -> Sum/2
  LatSpdHoldFlag/1 -> Sum/1
  Sum2/1 -> Product/2
  LatSpdHoldFlag1/1 -> Product/1

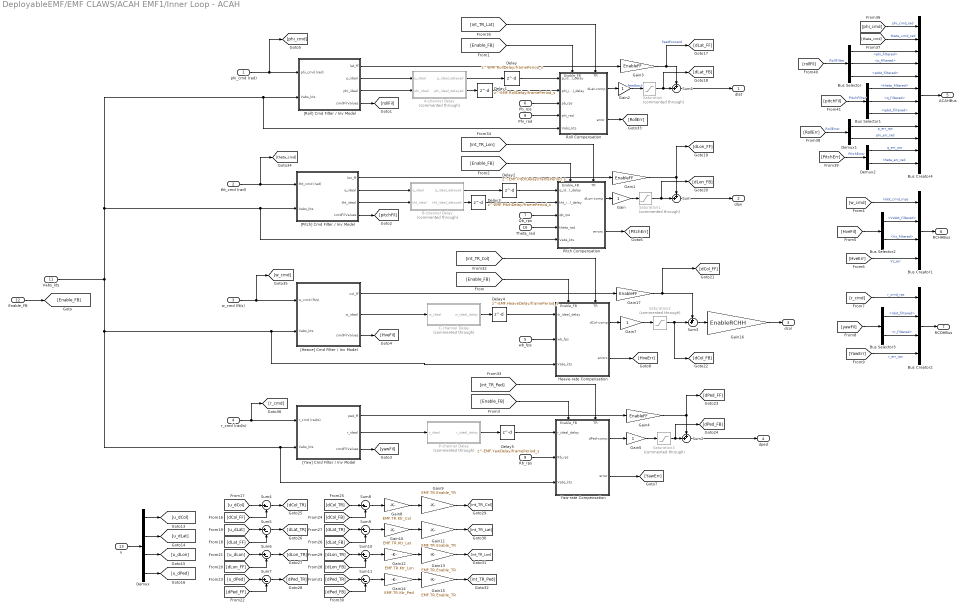
== system DeployableEMF/EMF CLAWS/ACAH EMF1/Inner Loop - ACAH ==
  phi_cmd (rad) : Inport
  tht_cmd (rad) : Inport  Port=2
  w_cmd (ft/s) : Inport  Port=3
  r_cmd (rad/s) : Inport  Port=4
  wb_fps : Inport  Port=5
  Pb_rps : Inport  Port=6
  Qb_rps : Inport  Port=7
  Rb_rps : Inport  Port=8
  Phi_rad : Inport  Port=9
  Theta_rad : Inport  Port=10
  Vabs_kts : Inport  Port=11
  Enable_FB : Inport  Port=12
  u : Inport  Port=13
  A-channel Delay : Subsystem  Commented=through
  B-channel Delay : Subsystem  Commented=through
  Bus Creator1 : BusCreator  Inputs=4
  Bus Creator2 : BusCreator  Inputs=4
  Bus Creator4 : BusCreator  Inputs=12
  Bus Selector : BusSelector  OutputSignals=phi_filtered,p_filtered,pdot_filtered
  Bus Selector1 : BusSelector  OutputSignals=theta_filtered,q_filtered,qdot_filtered
  Bus Selector2 : BusSelector  OutputSignals=Vzdot_filtered,Vz_filtered
  Bus Selector3 : BusSelector  OutputSignals=rdot_filtered,r_filtered
  C-channel Delay : Subsystem  Commented=through
  Delay : Delay  DelayLength=EMF.RollDelay/framePeriod_s
  Delay1 : Delay  DelayLength=EMF.RollDelay/framePeriod_s
  Delay2 : Delay  DelayLength=EMF.PitchDelay/framePeriod_s
  Delay3 : Delay  DelayLength=EMF.PitchDelay/framePeriod_s
  Delay4 : Delay  DelayLength=EMF.HeaveDelay/framePeriod_s
  Delay5 : Delay  DelayLength=EMF.YawDelay/framePeriod_s
  Demux : Demux
  Demux1 : Demux  Outputs=2
  Demux2 : Demux  Outputs=2
  Gain{,2,5,7} (4 alike) : Gain
  Gain{1,3..4,17} (4 alike) : Gain  Gain=EnableFF
  Gain10 : Gain  Gain=EMF.TR.Ktr_Lat
  Gain{9,11,13,15} (4 alike) : Gain  Gain=EMF.TR.Enable_TR
  Gain12 : Gain  Gain=EMF.TR.Ktr_Lon
  Gain14 : Gain  Gain=EMF.TR.Ktr_Ped
  Gain16 : Gain  Gain=EnableRCHH
  Gain8 : Gain  Gain=EMF.TR.Ktr_Col
  Heave-rate Compensation : Subsystem
      settings: PortSchema="{\"entries\":[{\"content\":{\"sides\":[{\"content\":{\"connectorIds\":[\"In1\",\"In2\",\"In3\"]},\"type\":\"ConnectorPlacement.EquallySpacedRectSide\",\"uuid\":\"7252c1f8-7fe3-4075-bb5e-c3f9f1883e70\"},{\"content\":{\"connectorIds\":[\"Out1\",\"Out2\"],\"side\":\"RIGHT\"},\"type\":\"ConnectorPlacement.EquallySpacedRectSide\",\"uuid\":\"3c35276a-72f6-40d6-83e0-8018ffb9b035\"},{\"content\":{\"connectorIds\":[\"In4\",\"In5\"],\"side\":\"TOP\"},\"type\":\"ConnectorPlacement.EquallySpacedRectSide\",\"uuid\":\"6ce22a11-3d6f-44d3-856f-73f158445266\"}]},\"type\":\"ConnectorPlacement.EquallySpacedConnector\",\"uuid\":\"443ffc0d-1192-4812-a7f7-f46c9ac66e90\"}],\"packageUris\":[\"http://schema.mathworks.com/mf0/Connector/R2020b\"],\"version\":\"1.0\"}"
  P-channel Delay : Subsystem  Commented=through
  Pitch Compensation : Subsystem
      settings: PortSchema="{\"entries\":[{\"content\":{\"sides\":[{\"content\":{\"connectorIds\":[\"In1\",\"In2\",\"In3\",\"In4\",\"In5\"]},\"type\":\"ConnectorPlacement.EquallySpacedRectSide\",\"uuid\":\"45916f42-37ac-4154-8414-b45309659ed0\"},{\"content\":{\"connectorIds\":[\"Out1\",\"Out2\"],\"side\":\"RIGHT\"},\"type\":\"ConnectorPlacement.EquallySpacedRectSide\",\"uuid\":\"89f52b07-9cdc-4229-907e-581f3d5d6e1b\"},{\"content\":{\"connectorIds\":[\"In6\",\"In7\"],\"side\":\"TOP\"},\"type\":\"ConnectorPlacement.EquallySpacedRectSide\",\"uuid\":\"5e1074eb-2cc8-4130-bee4-0f8c72f9550d\"}]},\"type\":\"ConnectorPlacement.EquallySpacedConnector\",\"uuid\":\"11c4fb04-7926-4153-b42d-1368c1a6596f\"}],\"packageUris\":[\"http://schema.mathworks.com/mf0/Connector/R2020b\"],\"version\":\"1.0\"}"
  Roll Compensation : Subsystem
      settings: PortSchema="{\"entries\":[{\"content\":{\"sides\":[{\"content\":{\"connectorIds\":[\"In1\",\"In2\",\"In3\",\"In4\",\"In5\"]},\"type\":\"ConnectorPlacement.EquallySpacedRectSide\",\"uuid\":\"45916f42-37ac-4154-8414-b45309659ed0\"},{\"content\":{\"connectorIds\":[\"Out1\",\"Out2\"],\"side\":\"RIGHT\"},\"type\":\"ConnectorPlacement.EquallySpacedRectSide\",\"uuid\":\"89f52b07-9cdc-4229-907e-581f3d5d6e1b\"},{\"content\":{\"connectorIds\":[\"In6\",\"In7\"],\"side\":\"TOP\"},\"type\":\"ConnectorPlacement.EquallySpacedRectSide\",\"uuid\":\"5e1074eb-2cc8-4130-bee4-0f8c72f9550d\"}]},\"type\":\"ConnectorPlacement.EquallySpacedConnector\",\"uuid\":\"11c4fb04-7926-4153-b42d-1368c1a6596f\"}],\"packageUris\":[\"http://schema.mathworks.com/mf0/Connector/R2020b\"],\"version\":\"1.0\"}"
  Saturation : Saturate  Commented=through  UpperLimit=EMF.MaxCmd.pdot/2  LowerLimit=-EMF.MaxCmd.pdot/2
  Saturation1 : Saturate  Commented=through  UpperLimit=EMF.MaxCmd.qdot/2  LowerLimit=-EMF.MaxCmd.qdot/2
  Saturation2 : Saturate  Commented=through  UpperLimit=EMF.MaxCmd.wdot/2  LowerLimit=-EMF.MaxCmd.wdot/2
  Saturation3 : Saturate  Commented=through  UpperLimit=EMF.MaxCmd.rdot/2  LowerLimit=-EMF.MaxCmd.rdot/2
  Sum{,1..3} (4 alike) : Sum  Inputs=++|
  Sum{4..11} (8 alike) : Sum  Inputs=|+-
  Yaw-rate Compensation : Subsystem
      settings: PortSchema="{\"entries\":[{\"content\":{\"sides\":[{\"content\":{\"connectorIds\":[\"In1\",\"In2\",\"In3\"]},\"type\":\"ConnectorPlacement.EquallySpacedRectSide\",\"uuid\":\"7252c1f8-7fe3-4075-bb5e-c3f9f1883e70\"},{\"content\":{\"connectorIds\":[\"Out1\",\"Out2\"],\"side\":\"RIGHT\"},\"type\":\"ConnectorPlacement.EquallySpacedRectSide\",\"uuid\":\"3c35276a-72f6-40d6-83e0-8018ffb9b035\"},{\"content\":{\"connectorIds\":[\"In4\",\"In5\"],\"side\":\"TOP\"},\"type\":\"ConnectorPlacement.EquallySpacedRectSide\",\"uuid\":\"6ce22a11-3d6f-44d3-856f-73f158445266\"}]},\"type\":\"ConnectorPlacement.EquallySpacedConnector\",\"uuid\":\"443ffc0d-1192-4812-a7f7-f46c9ac66e90\"}],\"packageUris\":[\"http://schema.mathworks.com/mf0/Connector/R2020b\"],\"version\":\"1.0\"}"
  "[Heave] Cmd Filter / Inv Model" : Subsystem
  "[Pitch] Cmd Filter / Inv Model" : Subsystem
  "[Roll] Cmd Filter / Inv Model" : Subsystem
  "[Yaw] Cmd Filter / Inv Model" : Subsystem
  dlat : Outport
  dlon : Outport  Port=2
  dcol : Outport  Port=3
  dped : Outport  Port=4
  ACAHBus : Outport  Port=5
  RCHHBus : Outport  Port=6
  RCDHBus : Outport  Port=7
  wires:
  Gain17/1 -> [dCol_FF], Sum3/1
  Gain5/1 -> Saturation3/1
  Gain4/1 -> Sum2/1, [dPed_FF]
  Gain3/1 -> [dLat_FF], Sum1/1  "feedforward"
  Gain2/1 -> Saturation/1  "feedback"
  Gain1/1 -> [dLon_FF], Sum/1
  Gain/1 -> Saturation1/1
  wb_fps/1 -> Heave-rate Compensation/2(wb_fps)
  Rb_rps/1 -> Yaw-rate Compensation/2(Rb_rps)
  Theta_rad/1 -> Pitch Compensation/4(theta_rad)
  Qb_rps/1 -> Pitch Compensation/3(qb_rps)
  Phi_rad/1 -> Roll Compensation/4(phi_rad)
  Pb_rps/1 -> Roll Compensation/3(pb_rps)
  "[Roll] Cmd Filter / Inv Model"/1(lat_ff) -> Gain3/1
  Roll Compensation/1(dLat-comp) -> Gain2/1
  "[Pitch] Cmd Filter / Inv Model"/1(lon_ff) -> Gain1/1
  Pitch Compensation/1(dLon-comp) -> Gain/1
  w_cmd (ft/s)/1 -> [w_cmd], "[Heave] Cmd Filter / Inv Model"/1(w_cmd (ft/s))
  r_cmd (rad/s)/1 -> [r_cmd], "[Yaw] Cmd Filter / Inv Model"/1(r_cmd (rad/s))
  "[Yaw] Cmd Filter / Inv Model"/1(ped_ff) -> Gain4/1
  "[Heave] Cmd Filter / Inv Model"/1(col_ff) -> Gain17/1
  Yaw-rate Compensation/1(dPed-comp) -> Gain5/1
  Heave-rate Compensation/1(dCol-comp) -> Gain7/1
  Pitch Compensation/2(errors) -> [PitchErr]
  Yaw-rate Compensation/2(error) -> [YawErr]
  Heave-rate Compensation/2(errors) -> [HveErr]
  "[Heave] Cmd Filter / Inv Model"/3(cmdFilValues) -> [HveFil]
  "[Yaw] Cmd Filter / Inv Model"/3(cmdFilValues) -> [yawFil]
  "[Pitch] Cmd Filter / Inv Model"/4(cmdFilValues) -> [pitchFil]
  "[Roll] Cmd Filter / Inv Model"/4(cmdFilValues) -> [rollFil]
  C-channel Delay/1(w_ideal_delay) -> Delay4/1
  Sum3/1 -> Gain16/1
  "[Heave] Cmd Filter / Inv Model"/2(w_ideal) -> C-channel Delay/1(w_ideal)
  "[Yaw] Cmd Filter / Inv Model"/2(r_ideal) -> P-channel Delay/1(r_ideal)
  Sum2/1 -> dped/1
  P-channel Delay/1(r_ideal_delay) -> Delay5/1
  "[Roll] Cmd Filter / Inv Model"/3(phi_ideal) -> A-channel Delay/2(phi_ideal)
  Sum1/1 -> dlat/1
  "[Roll] Cmd Filter / Inv Model"/2(p_ideal) -> A-channel Delay/1(p_ideal)
  A-channel Delay/2(phi_ideal_delayed) -> Delay1/1
  A-channel Delay/1(p_ideal_delayed) -> Delay/1
  Sum/1 -> dlon/1
  B-channel Delay/2(tht_ideal_delayed) -> Delay3/1
  B-channel Delay/1(q_ideal_delayed) -> Delay2/1
  "[Pitch] Cmd Filter / Inv Model"/2(q_ideal) -> B-channel Delay/1(q_ideal)
  "[Pitch] Cmd Filter / Inv Model"/3(tht_ideal) -> B-channel Delay/2(tht_ideal)
  Vabs_kts/1 -> Heave-rate Compensation/3(Vabs_kts), "[Heave] Cmd Filter / Inv Model"/2(Vabs_kts), Yaw-rate Compensation/3(Vabs_kts), "[Yaw] Cmd Filter / Inv Model"/2(Vabs_kts), Pitch Compensation/5(Vabs_kts), "[Pitch] Cmd Filter / Inv Model"/2(Vabs_kts), Roll Compensation/5(Vabs_kts), "[Roll] Cmd Filter / Inv Model"/2(Vabs_kts)
  phi_cmd (rad)/1 -> [phi_cmd], "[Roll] Cmd Filter / Inv Model"/1(phi_cmd (rad))
  tht_cmd (rad)/1 -> [theta_cmd], "[Pitch] Cmd Filter / Inv Model"/1(tht_cmd (rad))
  Delay1/1 -> Roll Compensation/2(phi_ideal_delay)
  Delay/1 -> Roll Compensation/1(p_ideal_delay)
  Delay3/1 -> Pitch Compensation/2(tht_ideal_delay)
  Delay2/1 -> Pitch Compensation/1(q_ideal_delay)
  Delay4/1 -> Heave-rate Compensation/1(w_ideal_delay)
  Delay5/1 -> Yaw-rate Compensation/1(r_ideal_delay)
  Enable_FB/1 -> [Enable_FB]
  [Enable_FB] -> Heave-rate Compensation/4(Enable_FB)
  [Enable_FB] -> Roll Compensation/6(Enable_FB)
  [Enable_FB] -> Pitch Compensation/6(Enable_FB)
  [Enable_FB] -> Yaw-rate Compensation/4(Enable_FB)
  Gain7/1 -> Saturation2/1
  Saturation/1 -> [dLat_FB], Sum1/2
  Saturation1/1 -> [dLon_FB], Sum/2
  Saturation3/1 -> [dPed_FB], Sum2/2
  u/1 -> Demux/1
  Demux/1 -> [u_dCol]
  Demux/4 -> [u_dPed]
  Demux/3 -> [u_dLon]
  Demux/2 -> [u_dLat]
  [u_dCol] -> Sum4/1
  [dCol_FF] -> Sum4/2
  Sum4/1 -> [dCol_TR]
  Sum5/1 -> [dLat_TR]
  [dLat_FF] -> Sum5/2
  [u_dLat] -> Sum5/1
  [u_dLon] -> Sum6/1
  [dLon_FF] -> Sum6/2
  Sum6/1 -> [dLon_TR]
  Sum7/1 -> [dPed_TR]
  [dPed_FF] -> Sum7/2
  [u_dPed] -> Sum7/1
  Sum8/1 -> Gain8/1
  [dCol_FB] -> Sum8/2
  [dCol_TR] -> Sum8/1
  Gain8/1 -> Gain9/1
  Gain9/1 -> [int_TR_Col]
  Gain11/1 -> [int_TR_Lat]
  Gain10/1 -> Gain11/1
  [dLat_TR] -> Sum9/1
  [dLat_FB] -> Sum9/2
  Sum9/1 -> Gain10/1
  Sum10/1 -> Gain12/1
  [dLon_FB] -> Sum10/2
  [dLon_TR] -> Sum10/1
  Gain12/1 -> Gain13/1
  Gain13/1 -> [int_TR_Lon]
  Gain15/1 -> [int_TR_Ped]
  Gain14/1 -> Gain15/1
  [dPed_TR] -> Sum11/1
  [dPed_FB] -> Sum11/2
  Sum11/1 -> Gain14/1
  [int_TR_Col] -> Heave-rate Compensation/5(TR)
  [int_TR_Ped] -> Yaw-rate Compensation/5(TR)
  [int_TR_Lon] -> Pitch Compensation/7(TR)
  [int_TR_Lat] -> Roll Compensation/7(TR)
  Saturation2/1 -> [dCol_FB], Sum3/2
  Gain16/1 -> dcol/1
  Roll Compensation/2(error) -> [RollErr]
  Bus Creator4/1 -> ACAHBus/1
  [phi_cmd] -> Bus Creator4/1  "phi_cmd_rad"
  [theta_cmd] -> Bus Creator4/2  "theta_cmd_rad"
  [rollFil] -> Bus Selector/1  "RollFilter"
  [pitchFil] -> Bus Selector1/1  "PitchFilter"
  Bus Selector/2 -> Bus Creator4/4  "<p_filtered>"
  Bus Selector/1 -> Bus Creator4/3  "<phi_filtered>"
  Bus Selector/3 -> Bus Creator4/5  "<pdot_filtered>"
  Bus Selector1/1 -> Bus Creator4/6  "<theta_filtered>"
  Bus Selector1/2 -> Bus Creator4/7  "<q_filtered>"
  Bus Selector1/3 -> Bus Creator4/8  "<qdot_filtered>"
  [RollErr] -> Demux1/1  "RollError"
  [PitchErr] -> Demux2/1  "PitchError"
  Demux2/2 -> Bus Creator4/12  "theta_err_rad"
  Demux2/1 -> Bus Creator4/11  "q_err_rps"
  Demux1/1 -> Bus Creator4/9  "p_err_rps"
  Demux1/2 -> Bus Creator4/10  "phi_err_rad"
  Bus Creator1/1 -> RCHHBus/1
  [w_cmd] -> Bus Creator1/1  "hdot_cmd_mps"
  [HveFil] -> Bus Selector2/1
  Bus Selector2/2 -> Bus Creator1/3  "<Vz_filtered>"
  Bus Selector2/1 -> Bus Creator1/2  "<Vzdot_filtered>"
  [HveErr] -> Bus Creator1/4  "Vz_err"
  [YawErr] -> Bus Creator2/4  "r_err_rps"
  Bus Selector3/1 -> Bus Creator2/2  "<rdot_filtered>"
  Bus Selector3/2 -> Bus Creator2/3  "<r_filtered>"
  [yawFil] -> Bus Selector3/1
  [r_cmd] -> Bus Creator2/1  "r_cmd_rps"
  Bus Creator2/1 -> RCDHBus/1

== system DeployableEMF/EMF CLAWS/ACAH EMF1/Mixer ==
  ControlMoments : Inport
  Constant : Constant  Value=EMF.Mixer(:,:,1)
  Matrix Multiply : Product  Multiplication=Matrix(*)
  Rotor Speeds : Outport
  wires:
  Constant/1 -> Matrix Multiply/1
  ControlMoments/1 -> Matrix Multiply/2
  Matrix Multiply/1 -> Rotor Speeds/1  "Rotor Speeds"
